simulink model "MainStateFlow_Pacemaker_group11"  (R2023a)
settings: Solver=FixedStepAuto  StartTime=0.0  StopTime=10.0  FixedStep=1e-3  RelTol=1e-3  EnableMultiTasking=on
undefined symbols (not defined in the file): D0, D1, D10, D11, D12, D13, D2, D3, D4, D5, D6, D7, D8, D9, PTA0, PTA1, PTA2, PTB23, PTB9, PTC16, PTC17, PTC2, PTC3, PTC4, PTD0, PTD1, PTD2, PTD3
libraries: frdmk64flib x16
settings Model: ExtModeTrigDuration=5  Creator=faraa  LastModifiedBy=faraa
settings OptimizationCC: EnhancedBackFolding=on  PassReuseOutputArgsAs=Individual arguments  ZeroExternalMemoryAtStartup=off  ZeroInternalMemoryAtStartup=off  MaxStackSize=64  OptimizeBlockOrder=speed  DifferentSizesBufferReuse=on  OptimizationCustomize=off  EfficientTunableParamExpr=on
settings DebuggingCC: ParameterTunabilityLossMsg=error
settings HardwareCC: ProdBitPerPointer=32  ProdBitPerSizeT=32  ProdBitPerPtrDiffT=32  ProdLargestAtomicInteger=Long  ProdLargestAtomicFloat=Double  ProdWordSize=32  ProdHWDeviceType=ARM Compatible->ARM Cortex
settings SFSimCC: MATLABDynamicMemAlloc=off
settings RTWCC: Description=Embedded Coder  SystemTargetFile=ert.tlc  HardwareBoard=NXP FRDM-K64F  TLCOptions="-aInlineSetEventsForThisBaseRateFcn=TLC_FALSE -aSuppressMultiTaskScheduler=TLC_FALSE  -aRateBasedStepFcn=0"  TemplateMakefile=ert_default_tmf  Toolchain=GNU Tools for ARM Embedded Processors
settings CodeAppCC: ForceParamTrailComments=on  IgnoreCustomStorageClasses=off  OperatorAnnotations=on  SimulinkDataObjDesc=on  SFDataObjDesc=on  InsertBlockDesc=on
settings ERTTargetCC: ExtModeTransport=4  ExtModeMexFile=sendToCommService

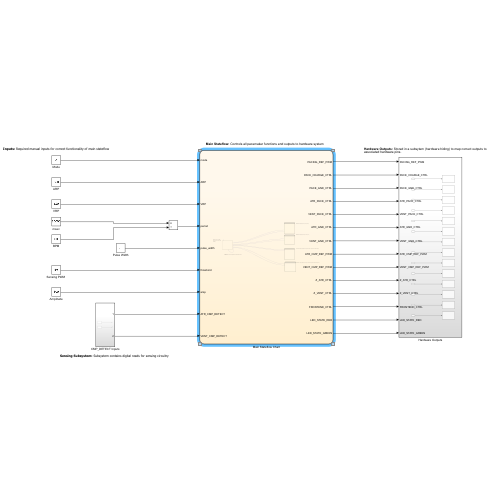
[thumbnail: Simulink's stored preview of the top-level diagram]
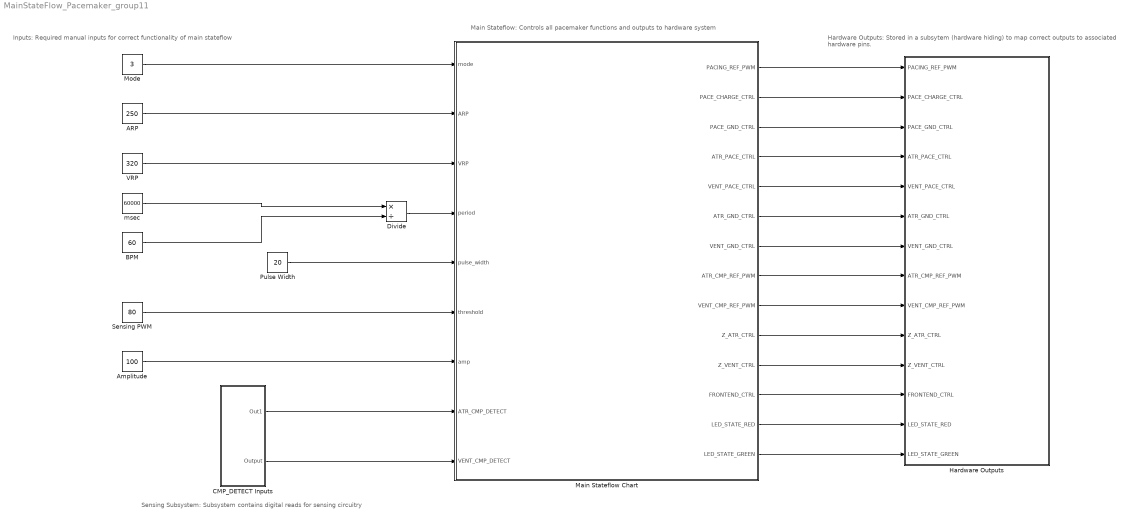
== system MainStateFlow_Pacemaker_group11 ==
  note: Inputs: Required manual inputs for correct functionality of main stateflow
  note: Sensing Subsystem: Subsystem contains digital reads for sensing circuitry
  note: Hardware Outputs: Stored in a subsytem (hardware hiding) to map correct outputs to associated hardware pins.
  note: Main Stateflow: Controls all pacemaker functions and outputs to hardware system
  ARP : Constant  Value=250
  Amplitude : Constant  Value=100
  BPM : Constant  Value=60
  CMP_DETECT Inputs : Subsystem
  Divide : Product  Inputs=*/
  Hardware Outputs : Subsystem
  Main Stateflow Chart : Stateflow chart  TreatAsAtomicUnit=on
  Mode : Constant  Value=3
  Pulse Width : Constant  Value=20
  "Sensing PWM " : Constant  Value=80
  VRP : Constant  Value=320
  msec : Constant  Value=60000
  wires:
  ARP/1 -> Main Stateflow Chart/2(ARP)
  VRP/1 -> Main Stateflow Chart/3(VRP)
  Divide/1 -> Main Stateflow Chart/4(period)
  Pulse Width/1 -> Main Stateflow Chart/5(pulse_width)
  Mode/1 -> Main Stateflow Chart/1(mode)
  "Sensing PWM "/1 -> Main Stateflow Chart/6(threshold)
  Amplitude/1 -> Main Stateflow Chart/7(amp)
  CMP_DETECT Inputs/1(Out1) -> Main Stateflow Chart/8(ATR_CMP_DETECT)
  CMP_DETECT Inputs/2(Output) -> Main Stateflow Chart/9(VENT_CMP_DETECT)
  msec/1 -> Divide/1
  BPM/1 -> Divide/2
  Main Stateflow Chart/1(PACING_REF_PWM) -> Hardware Outputs/1(PACING_REF_PWM)
  Main Stateflow Chart/2(PACE_CHARGE_CTRL) -> Hardware Outputs/2(PACE_CHARGE_CTRL)
  Main Stateflow Chart/4(ATR_PACE_CTRL) -> Hardware Outputs/4(ATR_PACE_CTRL)
  Main Stateflow Chart/6(ATR_GND_CTRL) -> Hardware Outputs/6(ATR_GND_CTRL)
  Main Stateflow Chart/10(Z_ATR_CTRL) -> Hardware Outputs/10(Z_ATR_CTRL)
  Main Stateflow Chart/7(VENT_GND_CTRL) -> Hardware Outputs/7(VENT_GND_CTRL)
  Main Stateflow Chart/5(VENT_PACE_CTRL) -> Hardware Outputs/5(VENT_PACE_CTRL)
  Main Stateflow Chart/11(Z_VENT_CTRL) -> Hardware Outputs/11(Z_VENT_CTRL)
  Main Stateflow Chart/8(ATR_CMP_REF_PWM) -> Hardware Outputs/8(ATR_CMP_REF_PWM)
  Main Stateflow Chart/9(VENT_CMP_REF_PWM) -> Hardware Outputs/9(VENT_CMP_REF_PWM)
  Main Stateflow Chart/13(LED_STATE_RED) -> Hardware Outputs/13(LED_STATE_RED)
  Main Stateflow Chart/14(LED_STATE_GREEN) -> Hardware Outputs/14(LED_STATE_GREEN)
  Main Stateflow Chart/12(FRONTEND_CTRL) -> Hardware Outputs/12(FRONTEND_CTRL)
  Main Stateflow Chart/3(PACE_GND_CTRL) -> Hardware Outputs/3(PACE_GND_CTRL)

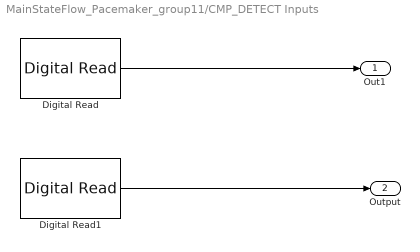
== system MainStateFlow_Pacemaker_group11/CMP_DETECT Inputs ==
  Digital Read : frdmk64flib/Digital Read  Whichpin=PTC16 (D0)  SampleTime=-1
  Digital Read1 : frdmk64flib/Digital Read  Whichpin=PTC17 (D1)  SampleTime=-1
  Out1 : Outport
  Output : Outport  Port=2
  wires:
  Digital Read/1 -> Out1/1
  Digital Read1/1 -> Output/1

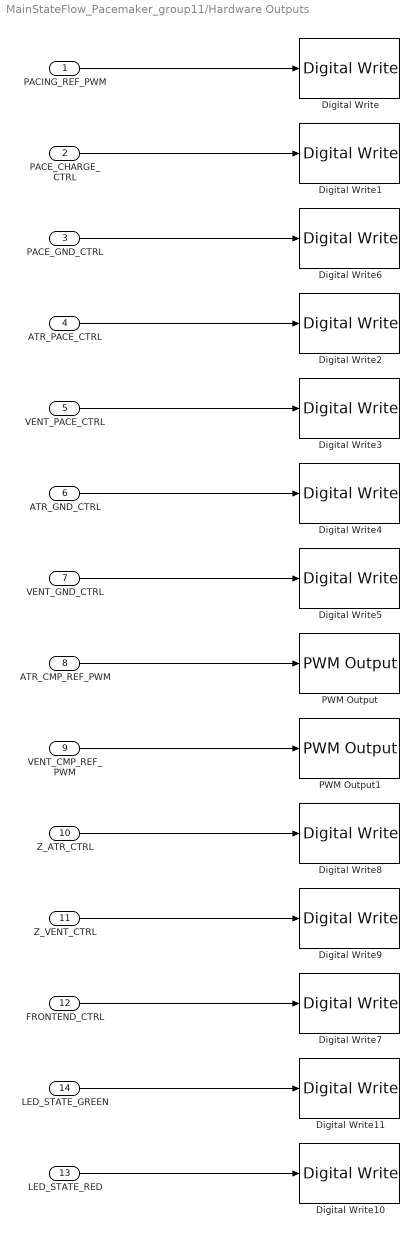
== system MainStateFlow_Pacemaker_group11/Hardware Outputs ==
  PACING_REF_PWM : Inport
  PACE_CHARGE_CTRL : Inport  Port=2
  PACE_GND_CTRL : Inport  Port=3
  ATR_PACE_CTRL : Inport  Port=4
  VENT_PACE_CTRL : Inport  Port=5
  ATR_GND_CTRL : Inport  Port=6
  VENT_GND_CTRL : Inport  Port=7
  ATR_CMP_REF_PWM : Inport  Port=8
  VENT_CMP_REF_PWM : Inport  Port=9
  Z_ATR_CTRL : Inport  Port=10
  Z_VENT_CTRL : Inport  Port=11
  FRONTEND_CTRL : Inport  Port=12
  LED_STATE_RED : Inport  Port=13
  LED_STATE_GREEN : Inport  Port=14
  Digital Write : frdmk64flib/Digital Write  Whichpin=PTA2 (D5)
  Digital Write1 : frdmk64flib/Digital Write  Whichpin=PTB9 (D2)
  Digital Write10 : frdmk64flib/Digital Write  Whichpin=RED_LED
  Digital Write11 : frdmk64flib/Digital Write  Whichpin=GREEN_LED
  Digital Write2 : frdmk64flib/Digital Write  Whichpin=PTA0 (D8)
  Digital Write3 : frdmk64flib/Digital Write  Whichpin=PTC4 (D9)
  Digital Write4 : frdmk64flib/Digital Write  Whichpin=PTD2 (D11)
  Digital Write5 : frdmk64flib/Digital Write  Whichpin=PTD3 (D12)
  Digital Write6 : frdmk64flib/Digital Write  Whichpin=PTD0 (D10)
  Digital Write7 : frdmk64flib/Digital Write  Whichpin=PTD1 (D13)
  Digital Write8 : frdmk64flib/Digital Write  Whichpin=PTB23 (D4)
  Digital Write9 : frdmk64flib/Digital Write  Whichpin=PTC3 (D7)
  PWM Output : frdmk64flib/PWM Output  Whichpin=PTC2 (D6)  InitialFrequency=2000  InitialDutyCycle=0
  PWM Output1 : frdmk64flib/PWM Output  Whichpin=PTA1 (D3)  InitialFrequency=2000  InitialDutyCycle=0
  wires:
  PACING_REF_PWM/1 -> Digital Write/1
  PACE_CHARGE_CTRL/1 -> Digital Write1/1
  ATR_PACE_CTRL/1 -> Digital Write2/1
  VENT_PACE_CTRL/1 -> Digital Write3/1
  ATR_GND_CTRL/1 -> Digital Write4/1
  VENT_GND_CTRL/1 -> Digital Write5/1
  ATR_CMP_REF_PWM/1 -> PWM Output/1
  VENT_CMP_REF_PWM/1 -> PWM Output1/1
  Z_ATR_CTRL/1 -> Digital Write8/1
  Z_VENT_CTRL/1 -> Digital Write9/1
  LED_STATE_RED/1 -> Digital Write10/1
  LED_STATE_GREEN/1 -> Digital Write11/1
  PACE_GND_CTRL/1 -> Digital Write6/1
  FRONTEND_CTRL/1 -> Digital Write7/1

== stateflow chart MainStateFlow_Pacemaker_group11/Main Stateflow Chart ==
  state AOO
    note: Charging: State to Charge C22 and discharge C21
        | and trigger LED indicators
    note: Pacing: Discharges C22 and charges C21
        | and triggers LED indicators
    state Pacing
      entry:
      PACE_CHARGE_CTRL=0;
      ATR_PACE_CTRL= 1;
      ATR_GND_CTRL= 0;
      PACE_GND_CTRL=1;
      LED_STATE_RED=false;
      LED_STATE_GREEN=true;
    state Charging
      entry:
      PACE_CHARGE_CTRL=1;
      ATR_PACE_CTRL= 0;
      ATR_GND_CTRL= 1;
      PACE_GND_CTRL=0;
      LED_STATE_RED=true;
      LED_STATE_GREEN=false;
    (default) -> AOO.Charging
    AOO.Charging -> AOO.Pacing : [after(period-pulse_width,msec)]
    AOO.Pacing -> AOO.Charging : [after(pulse_width,msec)]
  note: AOO: Performs charging and pacing for atrium (mode 0)
  state VOO
    note: Charging: State to Charge C22 and discharge C21
        | and trigger LED indicators
    note: Pacing: Discharges C22 and charges C21
        | and triggers LED indicators
    state Pacing
      entry:
      PACE_CHARGE_CTRL=0;
      VENT_PACE_CTRL= 1;
      VENT_GND_CTRL= 0;
      PACE_GND_CTRL=1;
      LED_STATE_RED=false;
      LED_STATE_GREEN=true;
    state Charging
      entry:
      PACE_CHARGE_CTRL = 1;
      VENT_PACE_CTRL = 0;
      VENT_GND_CTRL = 1;
      PACE_GND_CTRL = 0;
      LED_STATE_RED=true;
      LED_STATE_GREEN=false;
    (default) -> VOO.Charging
    VOO.Charging -> VOO.Pacing : [after(period-pulse_width,msec)]
    VOO.Pacing -> VOO.Charging : [after(pulse_width,msec)]
  note: VOO: Performs charging and pacing for ventricle (mode 1)
  note: Init: Initializes common variables
      | used throughout stateflow to reduce
      | redundancy
  state Init
    PACING_REF_PWM = amp;
    ATR_CMP_REF_PWM = threshold;
    VENT_CMP_REF_PWM = threshold;
    Z_VENT_CTRL = 0;
    Z_ATR_CTRL = 0;
    FRONTEND_CTRL = 0;
    LED_STATE_RED = false;
    LED_STATE_GREEN = false;
  state AAI
    note: Condition: Loops back to charging/sensing based on threshold detection
    state Pacing
      entry:
      PACE_CHARGE_CTRL = 0;
      ATR_PACE_CTRL = 1;
      ATR_GND_CTRL =0;
      PACE_GND_CTRL = 1;
      LED_STATE_RED = false;
      LED_STATE_GREEN = true;
    state Charging_Sensing
      %CHARGING
      entry:
      PACE_CHARGE_CTRL = 1;
      ATR_PACE_CTRL = 0;
      ATR_GND_CTRL =1;
      PACE_GND_CTRL = 0;
      %SENSING
      FRONTEND_CTRL = 1;
      LED_STATE_RED = true;
      LED_STATE_GREEN = false;
    note: Pacing: Discharges C22 and charges C21
        | and triggers LED indicators
    note: Charging: State to Charge C22 and discharge C21,
        | trigger LED indicators as well as implement sensing to determine when to pulse
    (junction 43) -> AAI.Charging_Sensing [order 1] : [ATR_CMP_DETECT == 1]
    (default) -> AAI.Charging_Sensing
    AAI.Charging_Sensing -> (junction 43) : [after(ARP-pulse_width,msec)]
    (junction 43) -> AAI.Pacing [order 2] : after(period-pulse_width,msec)[ATR_CMP_DETECT == 0]
    AAI.Pacing -> AAI.Charging_Sensing : [after(pulse_width,msec)]
  note: AAI: Performs charging, pacing and sensing for atrium based on a predetermined threshold (mode 2)
  note: Condition: Ensures no random output/behaviour if invalid modes are chosen
  state VVI
    note: Condition: Loops back to charging/sensing based on threshold detection
    state Pacing
      entry:
      PACE_CHARGE_CTRL = 0;
      VENT_PACE_CTRL = 1;
      VENT_GND_CTRL =0;
      PACE_GND_CTRL = 1;
      Z_VENT_CTRL =0;
      LED_STATE_RED = false;
      LED_STATE_GREEN = true;
    state Charging_Sensing
      %CHARGING
      entry:
      PACE_CHARGE_CTRL = 1;
      VENT_PACE_CTRL = 0;
      VENT_GND_CTRL =1;
      PACE_GND_CTRL = 0;
      %sSENSING
      FRONTEND_CTRL = 1;
      LED_STATE_RED = true;
      LED_STATE_GREEN = false;
    note: Pacing: Discharges C22 and charges C21
        | and triggers LED indicators
    note: Charging: State to Charge C22 and discharge C21,
        | trigger LED indicators as well as implement sensing to determine when to pulse
    (junction 59) -> VVI.Charging_Sensing [order 1] : [VENT_CMP_DETECT == 1]
    (default) -> VVI.Charging_Sensing
    (junction 59) -> VVI.Pacing [order 2] : after(period-pulse_width,msec)[VENT_CMP_DETECT == 0]
    VVI.Charging_Sensing -> (junction 59) : [after(VRP-pulse_width,msec)]
    VVI.Pacing -> VVI.Charging_Sensing : [after(pulse_width,msec)]
  note: VVI: Performs charging, pacing and sensing for ventricle based on a predetermined threshold (mode 3)
  Init -> AOO [order 1] : [mode==0]
  AOO -> Init : [mode ~= 0]
  Init -> VOO [order 2] : [mode == 1]
  (default) -> Init
  VOO -> Init : [mode ~= 1]
  Init -> AAI [order 3] : [mode == 2]
  AAI -> Init : [mode ~= 2]
  Init -> VVI [order 4] : [mode == 3]
  VVI -> Init : [mode ~= 3]
  Init -> Init [order 5] : [mode ~= 0 | mode ~=1 | mode ~= 2 | mode ~= 3]
  data: mode input; ARP input; VRP input; period input; pulse_width input; threshold input; amp input; ATR_CMP_DETECT input; VENT_CMP_DETECT input; PACING_REF_PWM output; PACE_CHARGE_CTRL output; PACE_GND_CTRL output; ATR_PACE_CTRL output; VENT_PACE_CTRL output; ATR_GND_CTRL output; VENT_GND_CTRL output; ATR_CMP_REF_PWM output; VENT_CMP_REF_PWM output; Z_ATR_CTRL output; Z_VENT_CTRL output; FRONTEND_CTRL output; LED_STATE_RED output; LED_STATE_GREEN output
